simulink model "IA1_final"  (R2022b)
settings: Solver=FixedStepAuto  StartTime=0.0  StopTime=5  FixedStep=0.1  RelTol=1e-3
libraries: simulink x2, simulink_extras x1
settings Model: Creator=Ccm  LastModifiedBy=Ccm
settings SolverCC: ZeroCrossControl=EnableAll  EnableFixedStepZeroCrossing=on

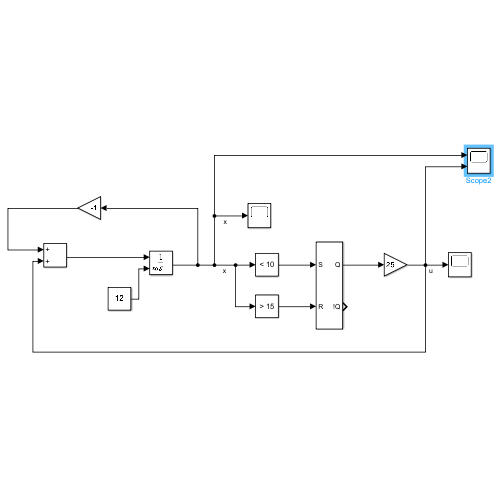
[thumbnail: Simulink's stored preview of the top-level diagram]
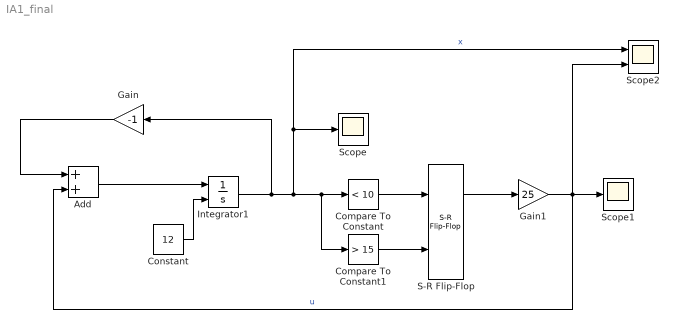
== system IA1_final ==
  Add : Sum
  Compare To Constant : simulink/Logic and Bit Operations/Compare To Constant  relop=<  const=10  OutDataTypeStr=boolean
  Compare To Constant1 : simulink/Logic and Bit Operations/Compare To Constant  relop=>  const=15  OutDataTypeStr=boolean
  Constant : Constant  Value=12
  Gain : Gain  Gain=-1
  Gain1 : Gain  Gain=25
  Integrator1 : Integrator  InitialConditionSource=external
  S-R Flip-Flop : simulink_extras/Flip Flops/S-R Flip-Flop  initial_condition=0
  Scope : Scope
  Scope1 : Scope
  Scope2 : Scope  NumInputPorts=2
  wires:
  S-R Flip-Flop/1 -> Gain1/1
  Gain1/1 -> Scope2/2, Add/2, Scope1/1  "u"
  Gain/1 -> Add/1
  Constant/1 -> Integrator1/2
  Add/1 -> Integrator1/1
  Integrator1/1 -> Gain/1, Scope2/1, Scope/1, Compare To Constant1/1, Compare To Constant/1  "x"
  Compare To Constant/1 -> S-R Flip-Flop/1
  Compare To Constant1/1 -> S-R Flip-Flop/2
